simulink model "Mazesolving"  (R2023a)
settings: Solver=FixedStepDiscrete  StartTime=0.0  StopTime=inf  FixedStep=0.01  RelTol=1e-3  EnableMultiTasking=on
undefined symbols (not defined in the file or in its folder): InputPWM, WheelSpeed
libraries: arduinolib x10, simulink x3, mobileRoboticsTrainingLib x1, arduinosensorlib x1
settings Model: ExtModeTrigDuration=2  Creator=thuto  LastModifiedBy=Nicola
settings OptimizationCC: EnhancedBackFolding=on  PassReuseOutputArgsAs=Individual arguments  ZeroExternalMemoryAtStartup=off  ZeroInternalMemoryAtStartup=off  MaxStackSize=64  OptimizeBlockOrder=speed  DifferentSizesBufferReuse=on  OptimizationCustomize=off  EfficientTunableParamExpr=on
settings DebuggingCC: ParameterTunabilityLossMsg=error
settings HardwareCC: ProdBitPerPointer=32  ProdBitPerSizeT=32  ProdBitPerPtrDiffT=32  ProdLargestAtomicInteger=Long  ProdLargestAtomicFloat=Double  ProdWordSize=32  ProdHWDeviceType=ARM Compatible->ARM Cortex  UseEmbeddedCoderFeatures=off  UseSimulinkCoderFeatures=off
settings SFSimCC: MATLABDynamicMemAlloc=off
settings RTWCC: Description=Embedded Coder  SystemTargetFile=ert.tlc  HardwareBoard=Arduino Nano 33 IoT  TemplateMakefile=ert_default_tmf  Toolchain=Arduino ARM  BuildConfiguration=Faster Runs
settings CodeAppCC: ForceParamTrailComments=on  IgnoreCustomStorageClasses=off  OperatorAnnotations=on  SimulinkDataObjDesc=on  SFDataObjDesc=on  InsertBlockDesc=on
settings ERTTargetCC: SupportContinuousTime=on  SupportNonInlinedSFcns=on  SupportVariableSizeSignals=on  ExtModeTransport=3  ExtModeStaticAlloc=on  ExtModeAutomaticAllocSize=off  ExtModeStaticAllocSize=8192  ExtModeMexFile=ext_xcp  ExtModeIntrfLevel=Level2 - Open

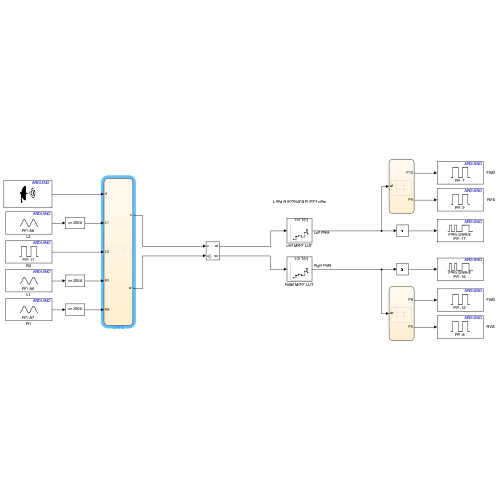
[thumbnail: Simulink's stored preview of the top-level diagram]
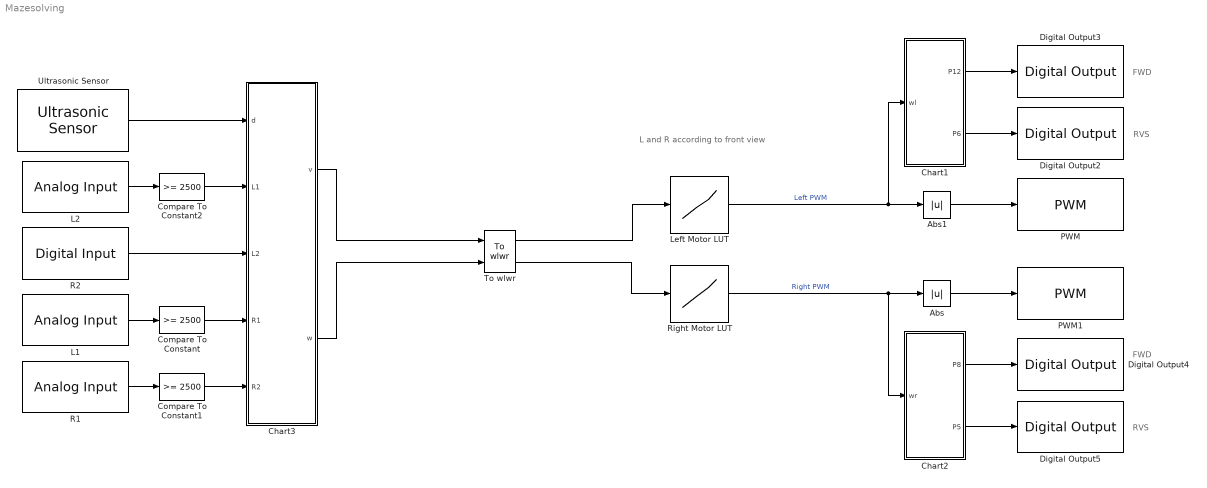
== system Mazesolving ==
  note: L and R according to front view
  note: FWD
  note: FWD
  note: RVS
  note: RVS
  Abs : Abs  SaturateOnIntegerOverflow=off
  Abs1 : Abs  SaturateOnIntegerOverflow=off
  Chart1 : Stateflow chart  TreatAsAtomicUnit=on
  Chart2 : Stateflow chart  TreatAsAtomicUnit=on
  Chart3 : Stateflow chart  TreatAsAtomicUnit=on
  Compare To Constant : simulink/Logic and Bit Operations/Compare To Constant  relop=>=  const=2500  OutDataTypeStr=boolean
  Compare To Constant1 : simulink/Logic and Bit Operations/Compare To Constant  relop=>=  const=2500  OutDataTypeStr=boolean
  Compare To Constant2 : simulink/Logic and Bit Operations/Compare To Constant  relop=>=  const=2500  OutDataTypeStr=boolean
  Digital Output2 : arduinolib/Digital Output  pinNumber=5  Direction=output  blockPlatform=arduino
  Digital Output3 : arduinolib/Digital Output  pinNumber=7  Direction=output  blockPlatform=arduino
  Digital Output4 : arduinolib/Digital Output  pinNumber=12  Direction=output  blockPlatform=arduino
  Digital Output5 : arduinolib/Digital Output  pinNumber=8  Direction=output  blockPlatform=arduino
  L1 : arduinolib/Analog Input  pinNumber=0  ReadResultsOnly=off  ConversionTriggerSource=Software  ExternalTriggerType=uint32( 0 )  OutputDataType=uint16  EnableConversionCompleteNotify=off  EnableOuputStatus=off  SampleTime=0.01  blockPlatform=arduino
  L2 : arduinolib/Analog Input  pinNumber=6  ReadResultsOnly=off  ConversionTriggerSource=Software  ExternalTriggerType=uint32( 0 )  OutputDataType=uint16  EnableConversionCompleteNotify=off  EnableOuputStatus=off  SampleTime=0.01  blockPlatform=arduino
  Left Motor LUT : Lookup_n-D  NumberOfTableDimensions=1  BreakpointsForDimension1=WheelSpeed  Table=InputPWM  InterpMethod=Nearest  ExtrapMethod=Clip  InternalRulePriority=Speed  RndMeth=Simplest
  PWM : arduinolib/PWM  pinNumber=17  frequencyType=Default  desiredFrequency=490.2  achievableFrequency=490.2
  PWM1 : arduinolib/PWM  pinNumber=16  frequencyType=Default  desiredFrequency=490.2  achievableFrequency=490.2
  R1 : arduinolib/Analog Input  pinNumber=7  ReadResultsOnly=off  ConversionTriggerSource=Software  ExternalTriggerType=uint32( 0 )  OutputDataType=uint16  EnableConversionCompleteNotify=off  EnableOuputStatus=off  SampleTime=0.01  blockPlatform=arduino
  R2 : arduinolib/Digital Input  pinNumber=11  mode=Default  Direction=input  SampleTime=0.01  blockPlatform=arduino
  Right Motor LUT : Lookup_n-D  NumberOfTableDimensions=1  BreakpointsForDimension1=WheelSpeed  Table=InputPWM  InterpMethod=Nearest  ExtrapMethod=Clip  InternalRulePriority=Speed  RndMeth=Simplest
  To wlwr : mobileRoboticsTrainingLib/To wlwr  axleLength=0.136  wheelR=0.062
  Ultrasonic Sensor : arduinosensorlib/Ultrasonic Sensor  NumSignalPins=2  TrigPin=9  EchoPin=10  SignalPin=3  SampleTime_=0.01  blockPlatform=ARDUINO
  wires:
  Right Motor LUT/1 -> Chart2/1(wr), Abs/1  "Right PWM"
  Left Motor LUT/1 -> Chart1/1(wl), Abs1/1  "Left PWM"
  L2/1 -> Compare To Constant2/1
  R2/1 -> Chart3/3(L2)
  L1/1 -> Compare To Constant/1
  Compare To Constant/1 -> Chart3/4(R1)
  R1/1 -> Compare To Constant1/1
  Chart1/2(P6) -> Digital Output2/1
  Chart1/1(P12) -> Digital Output3/1
  Chart2/1(P8) -> Digital Output4/1
  Chart2/2(P5) -> Digital Output5/1
  Compare To Constant1/1 -> Chart3/5(R2)
  Ultrasonic Sensor/1 -> Chart3/1(d)
  Abs/1 -> PWM1/1
  Abs1/1 -> PWM/1
  To wlwr/2 -> Right Motor LUT/1
  To wlwr/1 -> Left Motor LUT/1
  Compare To Constant2/1 -> Chart3/2(L1)
  Chart3/1(v) -> To wlwr/1
  Chart3/2(w) -> To wlwr/2

== stateflow chart Mazesolving/Chart1 ==
  state leftWheel
    (default) -> (junction 3)
    (junction 3) -> (junction 5) [order 1] : [wl>0]
    (junction 5) -> (junction 9) : {P12=1, P6=0;}
    (junction 3) -> (junction 12) [order 2] : {P12=0, P6=1;}
    (junction 9) -> (junction 12)
    (junction 12) -> (junction 15)
  (default) -> leftWheel
  data: wl input; P12 output; P6 output

== stateflow chart Mazesolving/Chart2 ==
  state rightWheel
    (default) -> (junction 3)
    (junction 3) -> (junction 5) [order 1] : [wr>0]
    (junction 5) -> (junction 9) : {P8=1, P5=0;}
    (junction 3) -> (junction 12) [order 2] : {P8=0, P5=1;}
    (junction 9) -> (junction 12)
    (junction 12) -> (junction 15)
  (default) -> rightWheel
  data: wr input; P8 output; P5 output

== stateflow chart Mazesolving/Chart3 ==
  state mazeSolving
    entry:
    n=0;
    closest=0;
    objects=zeros(5);
    vDef=0.4;
    wDef=6
    branch=0;
    wait=0.1;
    state testIntersection
      entry:
      turn=0;
      state branch [commented out]
        state branch [commented out]
          entry:
          n=n+1;
        state leftBranch [commented out]
          entry:
          branch=1;
        state rightBranch [commented out]
          entry:
          branch=-1;
        (default) -> mazeSolving.testIntersection.branch.branch [commented out]
        mazeSolving.testIntersection.branch.branch -> leftBranch [commented out] : [L2==0]
        mazeSolving.testIntersection.branch.branch -> rightBranch [commented out] : [R2==0]
      state turn90
        entry:
        v=0;
        w=10;
        state startTurn [commented out]
          entry:
          w=6;
          v=0;
        state right [commented out]
          entry:
          w=-wDef;
          v=0;
        state left [commented out]
          entry:
          w=wDef;
          v=0;
        state endTurn [commented out]
          entry:
          w=0;
          v=0;
        (default) -> mazeSolving.testIntersection.turn90.startTurn [commented out]
        mazeSolving.testIntersection.turn90.startTurn -> right [commented out] : [0==0]
        mazeSolving.testIntersection.turn90.startTurn -> left [commented out] : [0==1]
        right -> mazeSolving.testIntersection.turn90.endTurn [commented out] : [after(3, sec)]
      state goStraight
        entry:
        w=0;
        v=0.01;
      state stop
        entry:
        w=0;
        v=0;
      state end [commented out]
        entry:
        ending=1;
      mazeSolving.testIntersection.stop -> mazeSolving.testIntersection.branch [commented out] : [0==1]
      mazeSolving.testIntersection.branch -> mazeSolving.testIntersection.turn90 [commented out] : [branch~=0]
      (default) -> mazeSolving.testIntersection.goStraight
      mazeSolving.testIntersection.stop -> mazeSolving.testIntersection.turn90 : after(1, sec)
      mazeSolving.testIntersection.goStraight -> mazeSolving.testIntersection.stop : after(0.1, sec)
      mazeSolving.testIntersection.stop -> end [commented out] : [0==1]
    state lineFollowing
      state goCW
        entry:
        w=-wDef;
        v=0.8*vDef;
      state goStraight
        entry:
        w=0;
        v=vDef;
      state goCCW
        entry:
        w=wDef;
        v=0.8*vDef;
      (default) -> mazeSolving.lineFollowing.goStraight
      mazeSolving.lineFollowing.goCW -> mazeSolving.lineFollowing.goStraight : [L1==0]
      mazeSolving.lineFollowing.goCCW -> mazeSolving.lineFollowing.goStraight : [R1==0]
      mazeSolving.lineFollowing.goStraight -> mazeSolving.lineFollowing.goCW [order 2] : [L1==1]
      mazeSolving.lineFollowing.goStraight -> mazeSolving.lineFollowing.goCCW [order 1] : [R1==1]
    state detect [commented out]
      state stop [commented out]
        entry:
        w=0;
        v=0;
      state turn180 [commented out]
        entry:
        turn=0;
        state startTurn [commented out]
          entry:
          w=-wDef;
          v=0;
        state endTurn [commented out]
          entry:
          w=0;
          turn=1
        (default) -> mazeSolving.detect.turn180.startTurn [commented out]
        mazeSolving.detect.turn180.startTurn -> (junction 165) [commented out] : [L1==1 && R1==1]
        (junction 165) -> mazeSolving.detect.turn180.endTurn [commented out] : [L1==0 && R1==0]
      state measure [commented out]
        entry:
        objects(n)=d;
        (default) -> (junction 180) [commented out]
        (junction 180) -> (junction 176) [commented out] : [n==1 || d<objects(n-1)]
        (junction 180) -> (junction 184) [commented out] : {closest=closest}
        (junction 176) -> (junction 189) [commented out] : {closest=n}
        (junction 189) -> (junction 184) [commented out]
        (junction 184) -> (junction 190) [commented out]
      (default) -> mazeSolving.detect.stop [commented out]
      mazeSolving.detect.stop -> mazeSolving.detect.turn180 [commented out] : [L2==1 && R2==1]
      mazeSolving.detect.stop -> measure [commented out] : [L2==0 && R2==0]
      measure -> mazeSolving.detect.turn180 [commented out] : after(3, sec)
    state return [commented out]
      state turn180 [commented out]
        entry:
        turn=0;
        state startTurn [commented out]
          entry:
          w=-wDef;
          v=0;
        state endTurn [commented out]
          entry:
          w=0;
          turn=1
        (default) -> mazeSolving.return.turn180.startTurn [commented out]
        mazeSolving.return.turn180.startTurn -> (junction 259) [commented out] : [L1==1 && R1==1]
        (junction 259) -> mazeSolving.return.turn180.endTurn [commented out] : [L1==0 && R1==0]
      state lineFollowing [commented out]
        state goCW [commented out]
          entry:
          w=-wDef;
          v=vDef;
        state goStraight [commented out]
          entry:
          w = 0;
          v=vDef;
        state goCCW [commented out]
          entry:
          w=wDef;
          v=vDef;
        (default) -> mazeSolving.return.lineFollowing.goStraight [commented out]
        mazeSolving.return.lineFollowing.goCW -> mazeSolving.return.lineFollowing.goStraight [commented out] : [L1==0]
        mazeSolving.return.lineFollowing.goCCW -> mazeSolving.return.lineFollowing.goStraight [commented out] : [R1==0]
        mazeSolving.return.lineFollowing.goStraight -> mazeSolving.return.lineFollowing.goCW [commented out] : [L1==1]
        mazeSolving.return.lineFollowing.goStraight -> mazeSolving.return.lineFollowing.goCCW [commented out] : [R1==1]
      state stop [commented out]
        entry:
        w=0;
        v=0;
      state testIntersection [commented out]
        entry:
        turn=0;
        state countBranch [commented out]
          entry:
          n=n-1;
          turn=1;
        state branch [commented out]
          entry:
          branch=1;
        state turn90 [commented out]
          state startTurn [commented out]
            entry:
            v=0;
          state CW [commented out]
            during:
            w=-wDef;
          state CCW [commented out]
            during:
            w=wDef;
          state endTurn [commented out]
            entry:
            w=0;
            turn=1
          (default) -> mazeSolving.return.testIntersection.turn90.startTurn [commented out]
          mazeSolving.return.testIntersection.turn90.startTurn -> mazeSolving.return.testIntersection.turn90.CCW [commented out] : [R2==0]
          mazeSolving.return.testIntersection.turn90.startTurn -> mazeSolving.return.testIntersection.turn90.CW [commented out] : [L2==0]
          mazeSolving.return.testIntersection.turn90.CW -> (junction 314) [commented out] : [L1==1 && R1==1]
          mazeSolving.return.testIntersection.turn90.CCW -> (junction 314) [commented out] : [L1==1 && R1==1]
          (junction 314) -> mazeSolving.return.testIntersection.turn90.endTurn [commented out] : [L1==0 && R1==0]
        state goStraight [commented out]
          entry:
          w = 0;
          v=vDef;
        state stop [commented out]
          entry:
          w=0;
          v=0;
        (junction 307) -> countBranch [commented out] : [n>closest]
        (junction 307) -> mazeSolving.return.testIntersection.branch [commented out] : [n==closest]
        mazeSolving.return.testIntersection.branch -> mazeSolving.return.testIntersection.turn90 [commented out] : [branch~=0]
        mazeSolving.return.testIntersection.stop -> (junction 307) [commented out] : [L1==0 && R1==0]
        (default) -> mazeSolving.return.testIntersection.goStraight [commented out]
        mazeSolving.return.testIntersection.goStraight -> mazeSolving.return.testIntersection.stop [commented out] : after(1, sec)
        mazeSolving.return.testIntersection.stop -> mazeSolving.return.testIntersection.turn90 [commented out] : [L1==1 && R1==1]
      (default) -> mazeSolving.return.turn180 [commented out]
      mazeSolving.return.turn180 -> mazeSolving.return.lineFollowing [commented out] : [turn==1]
      mazeSolving.return.lineFollowing -> mazeSolving.return.stop [commented out] : [branch==1 && L1==1 && R1==1]
      mazeSolving.return.lineFollowing -> mazeSolving.return.testIntersection [commented out] : [xor(L2==0, R2==0) && branch==0]
      mazeSolving.return.testIntersection -> mazeSolving.return.lineFollowing [commented out] : [turn==1]
    state main [commented out]
      state goStraight [commented out]
        entry:
        w = 0;
        v=vDef;
      state startTurn [commented out]
        entry:
        v=0;
      state CW [commented out]
        during:
        w=-wDef;
      state CCW [commented out]
        during:
        w=wDef;
      state endTurn [commented out]
        entry:
        w=0;
        branch=0;
      (default) -> mazeSolving.main.goStraight [commented out]
      mazeSolving.main.goStraight -> mazeSolving.main.startTurn [commented out] : [L1==1 && R1==1]
      mazeSolving.main.startTurn -> mazeSolving.main.CW [commented out] : [branch==1]
      mazeSolving.main.startTurn -> mazeSolving.main.CCW [commented out] : [branch==-1]
      mazeSolving.main.CW -> (junction 209) [commented out] : [L1==1 && R1==1]
      mazeSolving.main.CCW -> (junction 209) [commented out] : [L1==1 && R1==1]
      (junction 209) -> mazeSolving.main.endTurn [commented out] : [L1==0 && R1==0]
    (default) -> mazeSolving.lineFollowing
    mazeSolving.lineFollowing -> mazeSolving.testIntersection : [L2==0 || R2==0]
    main -> mazeSolving.lineFollowing [commented out] : [branch==0]
    mazeSolving.lineFollowing -> detect [commented out] : [branch~=0 && L1==1 && R1==1]
    detect -> main [commented out] : [turn==1]
  (default) -> mazeSolving
  data: d input; v output; w output; closest local; objects local; n local; vDef local; L1 input; L2 input; R1 input; R2 input; turn local; branch local; ending local; wait local; wDef local
